simulink model "week2problem4"  (R2020b)
settings: Solver=VariableStepAuto  StartTime=0.0  StopTime=10.0  RelTol=1e-3
model workspace (MAT data in the model file):
  J = 3.2284e-06
  K = 0.0274
  L = 2.75e-06
  R = 4
  b = 3.5077e-06
settings Model: DataDictionary=problem4.sldd  OrderedModelArguments=off  Creator=Puru Gawande  LastModifiedBy=Puru Gawande

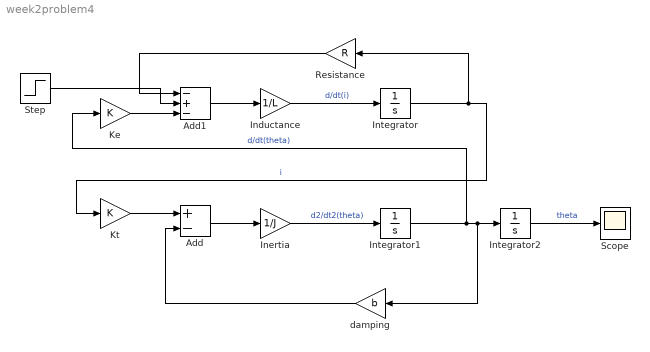
== system week2problem4 ==
  Add : Sum  Inputs=+-
  Add1 : Sum  Inputs=-+-
  Inductance : Gain  Gain=1/L
  Inertia : Gain  Gain=1/J
  Integrator : Integrator
  Integrator1 : Integrator
  Integrator2 : Integrator
  Ke : Gain  Gain=K
  Kt : Gain  Gain=K
  Resistance : Gain  Gain=R
  Scope : Scope
  Step : Step  SampleTime=0
  damping : Gain  Gain=b
  wires:
  Integrator1/1 -> Ke/1, Integrator2/1, damping/1  "d/dt(theta)"
  Step/1 -> Add1/2
  Integrator/1 -> Kt/1, Resistance/1  "i"
  Resistance/1 -> Add1/1
  Ke/1 -> Add1/3
  damping/1 -> Add/2
  Kt/1 -> Add/1
  Inertia/1 -> Integrator1/1  "d2/dt2(theta)"
  Inductance/1 -> Integrator/1  "d/dt(i)"
  Integrator2/1 -> Scope/1  "theta"
  Add1/1 -> Inductance/1
  Add/1 -> Inertia/1
